simulink model "sim_sistema_2_observador"  (Simulink 7.5)
settings: Solver=ode3  StartTime=0.0  StopTime=6  FixedStep=1e-4  RelTol=1e-3
values from neighbouring files (symbols this model uses):
  A = [0 1 0;0 0 1;-6 -11 -6;]    [exemplo10_8_b.m]
  Ac = Abb-Ke*Aab    [exemplo10_8_b.m]
  B = [0; 0; 1]    [exemplo10_8_b.m]
  Bc = Ac*Ke+Aba-Ke*Aaa    [exemplo10_8_b.m]
  Cc = [zeros(1,n-1);eye(n-1)]    [exemplo10_8_b.m]
  Dc = [1;Ke]    [exemplo10_8_b.m]
  Fc = Bb-Ke*Ba    [exemplo10_8_b.m]
  K = acker(A,B,J)    [exemplo10_8_b.m]
settings Model: Creator=taniel.franklin  LastModifiedBy=taniel.franklin

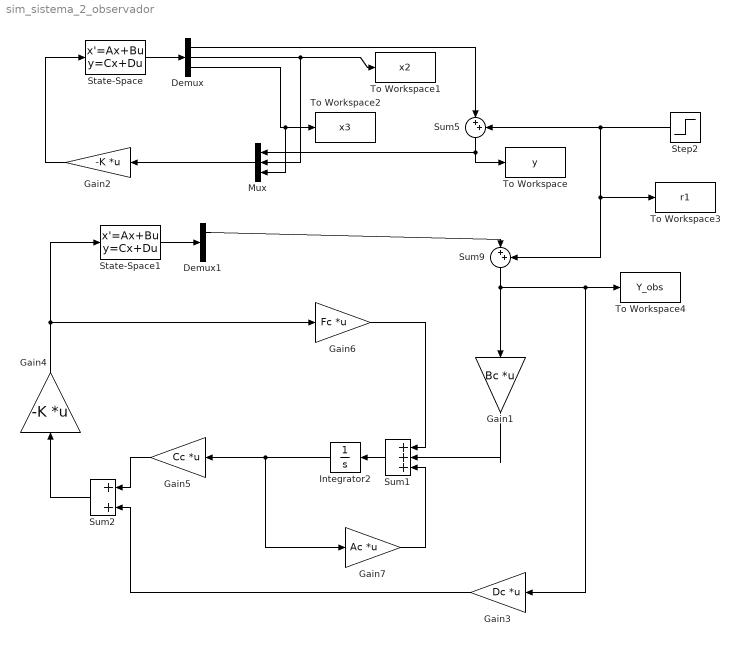
== system sim_sistema_2_observador ==
  Demux : Demux  Outputs=3
  Demux1 : Demux  Outputs=3
  Gain1 : Gain  Gain=Bc  Multiplication=Matrix(K*u)  ParameterDataType=fixdt(1, 16)  ParameterScaling=2^0  OutDataType=fixdt(1, 16)  OutScaling=2^0
  Gain2 : Gain  Gain=-K  Multiplication=Matrix(K*u)  ParameterDataType=fixdt(1, 16)  ParameterScaling=2^0  OutDataType=fixdt(1, 16)  OutScaling=2^0
  Gain3 : Gain  Gain=Dc  Multiplication=Matrix(K*u)  ParameterDataType=fixdt(1, 16)  ParameterScaling=2^0  OutDataType=fixdt(1, 16)  OutScaling=2^0
  Gain4 : Gain  Gain=-K  Multiplication=Matrix(K*u)  ParameterDataType=fixdt(1, 16)  ParameterScaling=2^0  OutDataType=fixdt(1, 16)  OutScaling=2^0
  Gain5 : Gain  Gain=Cc  Multiplication=Matrix(K*u)  ParameterDataType=fixdt(1, 16)  ParameterScaling=2^0  OutDataType=fixdt(1, 16)  OutScaling=2^0
  Gain6 : Gain  Gain=Fc  Multiplication=Matrix(K*u)  ParameterDataType=fixdt(1, 16)  ParameterScaling=2^0  OutDataType=fixdt(1, 16)  OutScaling=2^0
  Gain7 : Gain  Gain=Ac  Multiplication=Matrix(K*u)  ParameterDataType=fixdt(1, 16)  ParameterScaling=2^0  OutDataType=fixdt(1, 16)  OutScaling=2^0
  Integrator2 : Integrator
  Mux : Mux  Inputs=3
  State-Space : StateSpace  A=A  B=B  C=eye(3)  D=[0;0;0]
  State-Space1 : StateSpace  A=A  B=B  C=eye(3)  D=[0;0;0]
  Step2 : Step  Time=0.5  After=0.5  SampleTime=0
  Sum1 : Sum  Inputs=|+++  OutDataType=fixdt(1, 16)  OutScaling=2^0
  Sum2 : Sum  Inputs=|++  OutDataType=fixdt(1, 16)  OutScaling=2^0
  Sum5 : Sum  Inputs=|++  OutDataType=fixdt(1, 16)  OutScaling=2^0
  Sum9 : Sum  Inputs=|++  OutDataType=fixdt(1, 16)  OutScaling=2^0
  To Workspace : ToWorkspace  VariableName=y  SampleTime=-1  SaveFormat=Structure With Time
  To Workspace1 : ToWorkspace  VariableName=x2  SampleTime=-1  SaveFormat=Structure With Time
  To Workspace2 : ToWorkspace  VariableName=x3  SampleTime=-1  SaveFormat=Structure With Time
  To Workspace3 : ToWorkspace  VariableName=r1  SampleTime=-1  SaveFormat=Structure With Time
  To Workspace4 : ToWorkspace  VariableName=Y_obs  SampleTime=-1  SaveFormat=Structure With Time
  wires:
  State-Space/1 -> Demux/1
  Demux/2 -> To Workspace1/1, Mux/2
  Demux/3 -> To Workspace2/1, Mux/3
  Gain2/1 -> State-Space/1
  Demux/1 -> Sum5/1
  State-Space1/1 -> Demux1/1
  Sum5/1 -> To Workspace/1, Mux/1
  Step2/1 -> Sum5/2, Sum9/2, To Workspace3/1
  Demux1/1 -> Sum9/1
  Sum9/1 -> Gain1/1, To Workspace4/1, Gain3/1
  Gain6/1 -> Sum1/1
  Gain1/1 -> Sum1/2
  Integrator2/1 -> Gain7/1, Gain5/1
  Gain7/1 -> Sum1/3
  Sum1/1 -> Integrator2/1
  Gain3/1 -> Sum2/2
  Gain5/1 -> Sum2/1
  Sum2/1 -> Gain4/1
  Gain4/1 -> State-Space1/1, Gain6/1
  Mux/1 -> Gain2/1
